simulink model "ES239A_HwAgCorrln"  (R2013b)
settings: Solver=FixedStepDiscrete  SolverMode=SingleTasking  StartTime=0.0  StopTime=1  FixedStep=0.002  RelTol=1e-3
values from neighbouring files (symbols this model uses):
  FLTINJ_HWAGCORRLN_HWAGIDPTSIG = DataDict.Constant    [ES239A_HwAgCorrln_DataDict.m]
  HwAgCorrlnHwAgAbsltDif = DataDict.Calibration    [ES239A_HwAgCorrln_DataDict.m]
  HwAgCorrlnHwAgMaxStall = DataDict.Calibration    [ES239A_HwAgCorrln_DataDict.m]
  HwAgCorrlnNtc0x092FailStep = DataDict.Calibration    [ES239A_HwAgCorrln_DataDict.m]
  HwAgCorrlnNtc0x092PassStep = DataDict.Calibration    [ES239A_HwAgCorrln_DataDict.m]
undefined symbols (not defined in the file or in its folder): NtcNr1, NtcSts1, sigbuilder_block
libraries: simulink x2, NxtrLim x2
(part 1 of 2)
settings Model: Creator=rzqy0r  LastModifiedBy=FZG88Y
settings SolverCC: AutoInsertRateTranBlk=on  InsertRTBMode=Always
settings DataIOCC: LimitDataPoints=off  SaveFormat=Structure  ReturnWorkspaceOutputs=on
settings OptimizationCC: BlockReduction=off  InlineParams=on  ZeroExternalMemoryAtStartup=off  ZeroInternalMemoryAtStartup=off  OptimizeModelRefInitCode=on  LifeSpan=1
settings DebuggingCC: SignalInfNanChecking=error  SignalRangeChecking=warning  UnderspecifiedInitializationDetection=Simplified  SolverPrmCheckMsg=error  InheritedTsInSrcMsg=error  DiscreteInheritContinuousMsg=error  SingleTaskRateTransMsg=error  TasksWithSamePriorityMsg=error  SigSpecEnsureSampleTimeMsg=error  CheckMatrixSingularityMsg=error  ParameterUnderflowMsg=error  ParameterPrecisionLossMsg=error  ParameterTunabilityLossMsg=error  FixptConstUnderflowMsg=warning  FixptConstOverflowMsg=warning  VectorMatrixConversionMsg=error  SignalLabelMismatchMsg=error  UnconnectedInputMsg=error  UnconnectedOutputMsg=error  UnconnectedLineMsg=error  SFcnCompatibilityMsg=error  UniqueDataStoreMsg=warning  BusObjectLabelMismatch=error  RootOutportRequireBusObject=error  AssertControl=DisableAll  ModelReferenceIOMsg=error  ModelReferenceVersionMismatchMessage=warning  ModelReferenceIOMismatchMessage=error  ModelReferenceCSMismatchMessage=warning  ModelReferenceDataLoggingMessage=error  StateNameClashWarn=warning  StrictBusMsg=ErrorOnBusTreatedAsVector  NonBusSignalsTreatedAsBus=error  SFUnexpectedBacktrackingDiag=error  SFInvalidInputDataAccessInChartInitDiag=error  SFNoUnconditionalDefaultTransitionDiag=error  SFTransitionOutsideNaturalParentDiag=error  SFUnconditionalTransitionShadowingDiag=error  SFUndirectedBroadcastEventsDiag=error
settings ModelReferenceCC: ModelReferenceNumInstancesAllowed=Single
settings RTWCC: SystemTargetFile=autosar.tlc  GenCodeOnly=on  TemplateMakefile=ert_default_tmf  Description=AUTOSAR  GenerateReport=on  ProcessScript=autosar_make_rtw_hook  LaunchReport=on
settings CodeAppCC: GenerateComments=off  IgnoreCustomStorageClasses=off  CustomSymbolStrType=$N$R$M  CustomSymbolStrBlkIO=$N$M  SimulinkBlockComments=off
settings STFCustomTargetCC: ParMdlRefBuildCompliant=on  CompOptLevelCompliant=on  IncludeMdlTerminateFcn=off  CombineOutputUpdateFcns=on  SuppressErrorStatus=on  ERTFirstTimeCompliant=on  ERTCustomFileBanners=on  SupportNonFinite=off  SupportComplex=off  SupportContinuousTime=off  SupportNonInlinedSFcns=off  MATLABClassNameForMDSCustomization=Simulink.SoftwareTarget.ERTCustomization  AutosarCompliant=on  GRTInterface=off  SystemTargetFile=autosar.tlc
settings ERTTargetCC: CodeReplacementLibrary=ANSI_C  ConcurrentExecutionCompliant=off  IncludeMdlTerminateFcn=off  SuppressErrorStatus=on  SupportNonFinite=off  SupportComplex=off  ModelStepFunctionPrototypeControlCompliant=off  CPPClassGenCompliant=off  AutosarCompliant=on  InlinedParameterPlacement=NonHierarchical  ERTCustomFileTemplate=example_file_process.tlc  EnableUserReplacementTypes=on

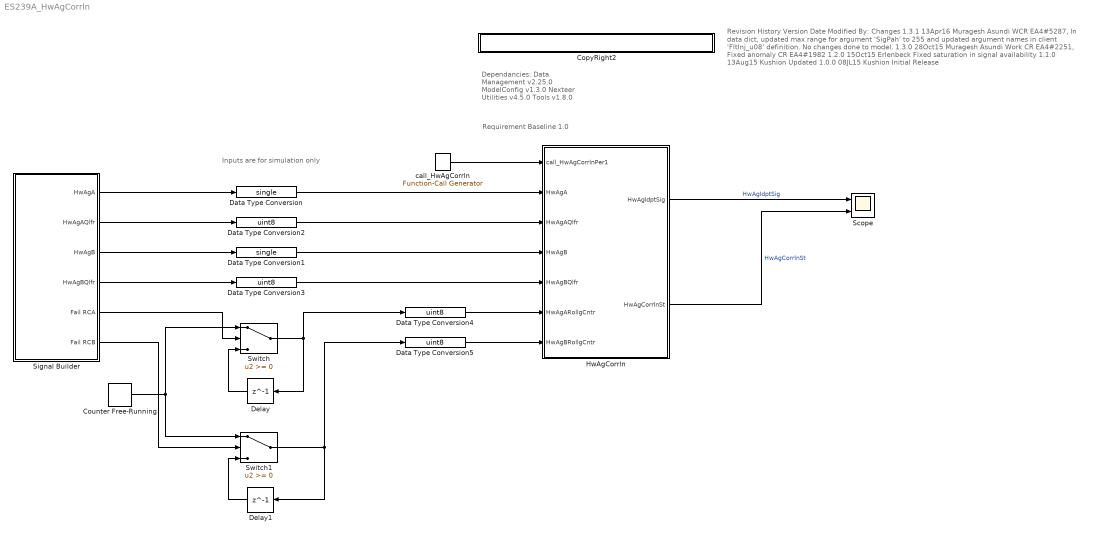
== system ES239A_HwAgCorrln ==
  note: Requirement Baseline 1.0
  note: Inputs are for simulation only
  note: Revision History
      |
      | Version		Date 		Modified By: 		Changes
      |
      | 1.3.1              13Apr16        Muragesh Asundi  WCR EA4#5287, In data dict, updated max range for argument 'SigPah' to 255 and updated argument names in client 'FltInj_u08' definition.
      |                                                                          No changes done to model.
      | 1.3.0              28Oct15        Muragesh Asundi  Work CR EA4#2251, Fixed anomaly CR EA4#1982
      | 1.2.0              15Oct15        Erlenbeck             Fixed saturation in signal availability
      | 1.1.0              13Aug15       Kushion                Updated
      | 1.0.0 		08JL15		Kushion			Initial Release
  note: Dependancies:
      |    Data Management v2.25.0
      |    ModelConfig v1.3.0
      |    Nexteer Utilities v4.5.0
      |    Tools v1.8.0
  CopyRight2 : Subsystem  Description=|  mask(Copyright Information){none=on}
      | Copyright info block.                                               
      |                                                                     
      | Place copyright information at the top of every subsystem in design.
      mask prompts: none "No parameters"
      mask help: Place copyright information at the top of every subsystem in design.
      mask Display:
      | NxtrConf = 'Nexteer Confidential';
      | 
      | sys = bdroot; %handle for the current model ("system")
      | first = get_param(sys,'Created');
      | first = first(end-3:end);  %year is last four digits
      | 
      | last = get_param(sys,'LastModifiedDate');
      | if isempty(last)
      |     last = datestr(now,'yyyy');
      | else
      |     last = last(end-3:end);
      | end
      | 
      | if strcmp(first,last)
      |     fprintf('%s -- Copyright %s Nexteer',NxtrConf,first)
      | else
      |     fprintf('%s -- %s%s- %s Nexteer',NxtrConf,char(169),first,last)
      | end
  Counter Free-Running : simulink/Sources/Counter Free-Running  NumBits=8  tsamp=0.004
  Data Type Conversion : DataTypeConversion  OutDataTypeStr=single
  Data Type Conversion1 : DataTypeConversion  OutDataTypeStr=single
  Data Type Conversion{2..5} (4 alike) : DataTypeConversion  OutDataTypeStr=uint8
  Delay : Delay  DelayLength=1  InitialCondition=0  SampleTime=0.004
  Delay1 : Delay  DelayLength=1  InitialCondition=0  SampleTime=0.004
  HwAgCorrln : Subsystem
      settings: AttributesFormatString=%<Tag>
  Scope : Scope  NumInputPorts=2
      settings: TimeRange=10  YMin=0~0  YMax=5~5  MaxDataPoints=10000
  Signal Builder : Subsystem  Tag=STV Subsys  LoadFcn=sigbuilder_block('load');  StartFcn=sigbuilder_block('start');  StopFcn=sigbuilder_block('stop');  ClipboardFcn=sigbuilder_block('clipboard');  mask(Sigbuilder block){}
      mask help: Simulink:masks:SigbuilderBlock_MD
      mask init:
      | if ~strcmp(get_param(bdroot(gcbh),'SimulationStatus'),'stopped') tuvar = sigbuilder_block('maskInit'); end
      settings: CopyFcn=sigbuilder_block('copy');  DeleteFcn=sigbuilder_block('delete');  ModelCloseFcn=sigbuilder_block('modelClose');  PreSaveFcn=sigbuilder_block('preSave');  PauseFcn=sigbuilder_block('pause');  ContinueFcn=sigbuilder_block('continue');  NameChangeFcn=sigbuilder_block('namechange');  OpenFcn=sigbuilder_block('open',[21.75 99 490.5 414 ]);  CloseFcn=sigbuilder_block('close');
      mask Display: plot(0, 0, 100, 100,[2, 2, 32, 32, 2], [68, 8, 8, 68, 68],[32, 2], [38, 38], [32, 19, 2],[53, 60, 44], [32, 17, 17, 2],[16, 16, 31, 31]);txt = getActiveGroup(gcbh);text(2, 100, txt,'verticalAlignment', 'top');
  Switch : Switch
  Switch1 : Switch
  call_HwAgCorrln : simulink/Ports & Subsystems/Function-Call Generator  sample_time=.004  numberOfIterations=1
  wires:
  call_HwAgCorrln/1 -> HwAgCorrln/1(call_HwAgCorrlnPer1)
  HwAgCorrln/1(HwAgIdptSig) -> Scope/1  "HwAgIdptSig"
  HwAgCorrln/2(HwAgCorrlnSt) -> Scope/2  "HwAgCorrlnSt"
  Signal Builder/5(Fail RCA) -> Switch/2
  Delay/1 -> Switch/3
  Switch/1 -> Delay/1, Data Type Conversion4/1
  Counter Free-Running/1 -> Switch1/1, Switch/1
  Signal Builder/6(Fail RCB) -> Switch1/2
  Delay1/1 -> Switch1/3
  Switch1/1 -> Data Type Conversion5/1, Delay1/1
  Signal Builder/1(HwAgA) -> Data Type Conversion/1
  Signal Builder/2(HwAgAQlfr) -> Data Type Conversion2/1
  Signal Builder/3(HwAgB) -> Data Type Conversion1/1
  Signal Builder/4(HwAgBQlfr) -> Data Type Conversion3/1
  Data Type Conversion1/1 -> HwAgCorrln/4(HwAgB)
  Data Type Conversion2/1 -> HwAgCorrln/3(HwAgAQlfr)
  Data Type Conversion3/1 -> HwAgCorrln/5(HwAgBQlfr)
  Data Type Conversion4/1 -> HwAgCorrln/6(HwAgARollgCntr)
  Data Type Conversion5/1 -> HwAgCorrln/7(HwAgBRollgCntr)
  Data Type Conversion/1 -> HwAgCorrln/2(HwAgA)

== system ES239A_HwAgCorrln/CopyRight2 ==

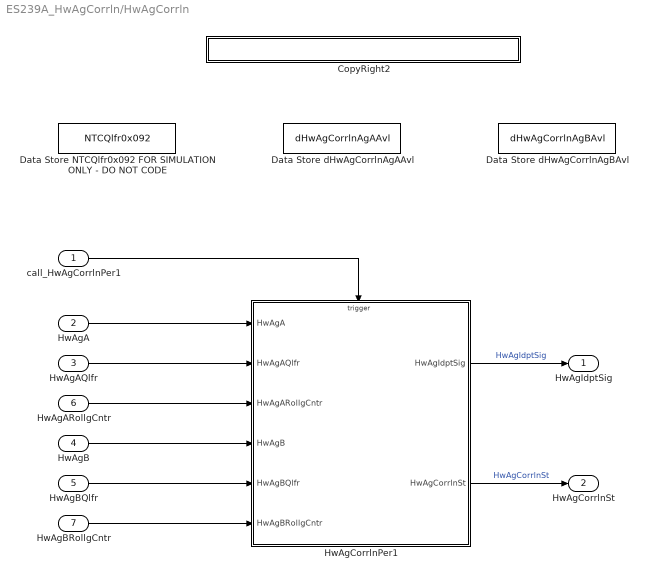
== system ES239A_HwAgCorrln/HwAgCorrln ==
  call_HwAgCorrlnPer1 : Inport
  HwAgA : Inport  Port=2
  HwAgAQlfr : Inport  Port=3
  HwAgB : Inport  Port=4
  HwAgBQlfr : Inport  Port=5
  HwAgARollgCntr : Inport  Port=6
  HwAgBRollgCntr : Inport  Port=7
  CopyRight2 : Subsystem  Description=|  mask(Copyright Information){none=on}
      | Copyright info block.                                               
      |                                                                     
      | Place copyright information at the top of every subsystem in design.
      mask prompts: none "No parameters"
      mask help: Place copyright information at the top of every subsystem in design.
      mask Display:
      | NxtrConf = 'Nexteer Confidential';
      | 
      | sys = bdroot; %handle for the current model ("system")
      | first = get_param(sys,'Created');
      | first = first(end-3:end);  %year is last four digits
      | 
      | last = get_param(sys,'LastModifiedDate');
      | if isempty(last)
      |     last = datestr(now,'yyyy');
      | else
      |     last = last(end-3:end);
      | end
      | 
      | if strcmp(first,last)
      |     fprintf('%s -- Copyright %s Nexteer',NxtrConf,first)
      | else
      |     fprintf('%s -- %s%s- %s Nexteer',NxtrConf,char(169),first,last)
      | end
  Data Store NTCQlfr0x092 FOR SIMULATION ONLY - DO NOT CODE : DataStoreMemory  DataStoreName=NTCQlfr0x092
  Data Store dHwAgCorrlnAgAAvl : DataStoreMemory  DataStoreName=dHwAgCorrlnAgAAvl
  Data Store dHwAgCorrlnAgBAvl : DataStoreMemory  DataStoreName=dHwAgCorrlnAgBAvl
  HwAgCorrlnPer1 : Subsystem  Tag=0.002  TreatAsAtomicUnit=on
  HwAgIdptSig : Outport
  HwAgCorrlnSt : Outport  Port=2
  wires:
  HwAgCorrlnPer1/1(HwAgIdptSig) -> HwAgIdptSig/1  "HwAgIdptSig"
  call_HwAgCorrlnPer1/1 -> HwAgCorrlnPer1/Trigger
  HwAgA/1 -> HwAgCorrlnPer1/1(HwAgA)
  HwAgAQlfr/1 -> HwAgCorrlnPer1/2(HwAgAQlfr)
  HwAgARollgCntr/1 -> HwAgCorrlnPer1/3(HwAgARollgCntr)
  HwAgB/1 -> HwAgCorrlnPer1/4(HwAgB)
  HwAgBQlfr/1 -> HwAgCorrlnPer1/5(HwAgBQlfr)
  HwAgBRollgCntr/1 -> HwAgCorrlnPer1/6(HwAgBRollgCntr)
  HwAgCorrlnPer1/2(HwAgCorrlnSt) -> HwAgCorrlnSt/1  "HwAgCorrlnSt"

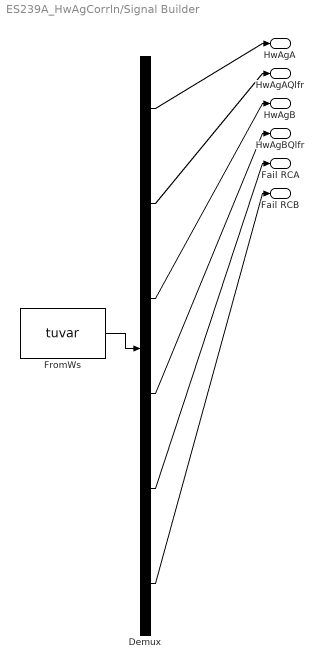
== system ES239A_HwAgCorrln/Signal Builder ==
  Demux : Demux  Tag=STV Demux  Outputs=6
  FromWs : FromWorkspace  Tag=STV FromWs  VariableName=tuvar  SampleTime=0
      SigBuilderData=|
      | common.afterFinalStr = 'Extrapolate'
      | common.sampleTime = 0
      | dataSet(1).timeRange = [0 10]
      | dataSet(1).name = 'Normal Op'
      | dataSet(2).timeRange = [0 10]
      | dataSet(2).name = 'Correlation Failure'
      | dataSet(3).timeRange = [0 10]
      | dataSet(3).name = 'Qualifier A Failure Hold Last Value with Recovery'
      | dataSet(4).timeRange = [0 10]
      | dataSet(4).name = 'Short Qualifier A Failure - Confirm immediate Status but no indpt reduction'
      | dataSet(5).timeRange = [0 10]
      | dataSet(5).name = 'Qualifier A and B Failure with recovery'
      | sbobj.Groups(1).Name = 'Normal Op'
      | sbobj.Groups(1).Signals(1).Name = 'HwAgA'
      | sbobj.Groups(1).Signals(1).XData = [0 1 2 3 4 5 6 7 8 9 10]
      | sbobj.Groups(1).Signals(1).YData = [0 900 -900 900 -900 900 -222 180 0 0 0]
      | sbobj.Groups(1).Signals(2).Name = 'HwAgAQlfr'
      | sbobj.Groups(1).Signals(2).XData = [0 0.8 0.8 6 10]
      | sbobj.Groups(1).Signals(2).YData = [0 0 1 1 1]
      | sbobj.Groups(1).Signals(3).Name = 'HwAgB'
      | sbobj.Groups(1).Signals(3).XData = [0 1 2 3 4 5 6 7 8 9 10]
      | sbobj.Groups(1).Signals(3).YData = [0 900 -900 900 -900 900 -222 180 0 0 0]
      | sbobj.Groups(1).Signals(4).Name = 'HwAgBQlfr'
      | sbobj.Groups(1).Signals(4).XData = [0 1 1 2 10]
      | sbobj.Groups(1).Signals(4).YData = [0 0 1 1 1]
      | sbobj.Groups(1).Signals(5).Name = 'Fail RCA'
      | sbobj.Groups(1).Signals(5).XData = [0 4 6 10]
      | sbobj.Groups(1).Signals(5).YData = [1 1 1 1]
      | sbobj.Groups(1).Signals(6).Name = 'Fail RCB'
      | sbobj.Groups(1).Signals(6).XData = [0 4 6 10]
      | sbobj.Groups(1).Signals(6).YData = [1 1 1 1]
      | sbobj.Groups(2).Name = 'Correlation Failure'
      | sbobj.Groups(2).Signals(1).Name = 'HwAgA'
      | sbobj.Groups(2).Signals(1).XData = [0 1 2 3 4 5 6 7 8 9 10]
      | sbobj.Groups(2).Signals(1).YData = [0 900 -900 900 -900 900 -222 180 0 0 0]
      | sbobj.Groups(2).Signals(2).Name = 'HwAgAQlfr'
      | sbobj.Groups(2).Signals(2).XData = [0 0.8 0.8 6 10]
      | sbobj.Groups(2).Signals(2).YData = [0 0 1 1 1]
      | sbobj.Groups(2).Signals(3).Name = 'HwAgB'
      | sbobj.Groups(2).Signals(3).XData = [0 1 2 3 4 5 6 7 8 9 10]
      | sbobj.Groups(2).Signals(3).YData = [0 900 -900 900 -900 900 -222 -264.9 0 0 0]
      | sbobj.Groups(2).Signals(4).Name = 'HwAgBQlfr'
      | sbobj.Groups(2).Signals(4).XData = [0 1 1 2 10]
      | sbobj.Groups(2).Signals(4).YData = [0 0 1 1 1]
      | sbobj.Groups(2).Signals(5).Name = 'Fail RCA'
      | sbobj.Groups(2).Signals(5).XData = [0 4 6 10]
      | sbobj.Groups(2).Signals(5).YData = [1 1 1 1]
      | sbobj.Groups(2).Signals(6).Name = 'Fail RCB'
      | sbobj.Groups(2).Signals(6).XData = [0 4 6 10]
      | sbobj.Groups(2).Signals(6).YData = [1 1 1 1]
      | sbobj.Groups(3).Name = 'Qualifier A Failure Hold Last Value with Recovery'
      | sbobj.Groups(3).Signals(1).Name = 'HwAgA'
      | sbobj.Groups(3).Signals(1).XData = [0 1 2 3 4 5 6 7 8 9 10]
      | sbobj.Groups(3).Signals(1).YData = [0 900 -900 900 -900 900 -222 180 0 0 0]
      | sbobj.Groups(3).Signals(2).Name = 'HwAgAQlfr'
      | sbobj.Groups(3).Signals(2).XData = [0 0.8 0.8 6 10]
      | sbobj.Groups(3).Signals(2).YData = [0 0 1 1 1]
      | sbobj.Groups(3).Signals(3).Name = 'HwAgB'
      | sbobj.Groups(3).Signals(3).XData = [0 1 2 3 4 5 5 6 7 8 9 10]
      | sbobj.Groups(3).Signals(3).YData = [0 900 -900 -900 -900 -900 900 -222 180 0 0 0]
      | sbobj.Groups(3).Signals(4).Name = 'HwAgBQlfr'
      | sbobj.Groups(3).Signals(4).XData = [0 1 1 2 2 3 4 5 5 10]
      | sbobj.Groups(3).Signals(4).YData = [0 0 1 1 2 2 2 2 1 1]
      | sbobj.Groups(3).Signals(5).Name = 'Fail RCA'
      | sbobj.Groups(3).Signals(5).XData = [0 4 6 10]
      | sbobj.Groups(3).Signals(5).YData = [1 1 1 1]
      | sbobj.Groups(3).Signals(6).Name = 'Fail RCB'
      | sbobj.Groups(3).Signals(6).XData = [0 4 6 10]
      | sbobj.Groups(3).Signals(6).YData = [1 1 1 1]
      | sbobj.Groups(4).Name = 'Short Qualifier A Failure - Confirm immediate Status but no indpt reduction'
      | sbobj.Groups(4).Signals(1).Name = 'HwAgA'
      | sbobj.Groups(4).Signals(1).XData = [0 1 2 3 4 5 6 7 8 9 10]
      | sbobj.Groups(4).Signals(1).YData = [0 900 -900 900 -900 900 -222 180 0 0 0]
      | sbobj.Groups(4).Signals(2).Name = 'HwAgAQlfr'
      | sbobj.Groups(4).Signals(2).XData = [0 0.8 0.8 6 10]
      | sbobj.Groups(4).Signals(2).YData = [0 0 1 1 1]
      | sbobj.Groups(4).Signals(3).Name = 'HwAgB'
      | sbobj.Groups(4).Signals(3).XData = [0 1 2 3 4 5 6 7 8 9 10]
      | sbobj.Groups(4).Signals(3).YData = [0 900 -900 900 -900 900 -222 180 0 0 0]
      | sbobj.Groups(4).Signals(4).Name = 'HwAgBQlfr'
      | sbobj.Groups(4).Signals(4).XData = [0 1 1 2 2 2.05 2.05 4 5 10]
      | sbobj.Groups(4).Signals(4).YData = [0 0 1 1 2 2 1 1 1 1]
      | sbobj.Groups(4).Signals(5).Name = 'Fail RCA'
      | sbobj.Groups(4).Signals(5).XData = [0 4 6 10]
      | sbobj.Groups(4).Signals(5).YData = [1 1 1 1]
      | sbobj.Groups(4).Signals(6).Name = 'Fail RCB'
      | sbobj.Groups(4).Signals(6).XData = [0 4 6 10]
      | sbobj.Groups(4).Signals(6).YData = [1 1 1 1]
      | sbobj.Groups(5).Name = 'Qualifier A and B Failure with recovery'
      | sbobj.Groups(5).Signals(1).Name = 'HwAgA'
      | sbobj.Groups(5).Signals(1).XData = [0 1 2 3 4 5 6 6 7 8 9 10]
      | sbobj.Groups(5).Signals(1).YData = [0 900 -900 900 -900 -900 -900 -222 180 0 0 0]
      | sbobj.Groups(5).Signals(2).Name = 'HwAgAQlfr'
      | sbobj.Groups(5).Signals(2).XData = [0 0.8 0.8 4 4 6 6 10]
      | sbobj.Groups(5).Signals(2).YData = [0 0 1 1 2 2 1 1]
      | sbobj.Groups(5).Signals(3).Name = 'HwAgB'
      | sbobj.Groups(5).Signals(3).XData = [0 1 2 3 4 5 5 6 7 8 9 10]
      | sbobj.Groups(5).Signals(3).YData = [0 900 -900 -900 -900 -900 900 -222 180 0 0 0]
      | sbobj.Groups(5).Signals(4).Name = 'HwAgBQlfr'
      | sbobj.Groups(5).Signals(4).XData = [0 1 1 2 2 3 4 5 5 10]
      | sbobj.Groups(5).Signals(4).YData = [0 0 1 1 2 2 2 2 1 1]
      | sbobj.Groups(5).Signals(5).Name = 'Fail RCA'
      | sbobj.Groups(5).Signals(5).XData = [0 4 6 10]
      | sbobj.Groups(5).Signals(5).YData = [1 1 1 1]
      | sbobj.Groups(5).Signals(6).Name = 'Fail RCB'
      | sbobj.Groups(5).Signals(6).XData = [0 4 6 10]
      | sbobj.Groups(5).Signals(6).YData = [1 1 1 1]
  HwAgA : Outport  Tag=STV Outport
  HwAgAQlfr : Outport  Tag=STV Outport  Port=2
  HwAgB : Outport  Tag=STV Outport  Port=3
  HwAgBQlfr : Outport  Tag=STV Outport  Port=4
  Fail RCA : Outport  Tag=STV Outport  Port=5
  Fail RCB : Outport  Tag=STV Outport  Port=6
  wires:
  FromWs/1 -> Demux/1
  Demux/1 -> HwAgA/1
  Demux/2 -> HwAgAQlfr/1
  Demux/3 -> HwAgB/1
  Demux/4 -> HwAgBQlfr/1
  Demux/5 -> Fail RCA/1
  Demux/6 -> Fail RCB/1

== system ES239A_HwAgCorrln/HwAgCorrln/CopyRight2 ==

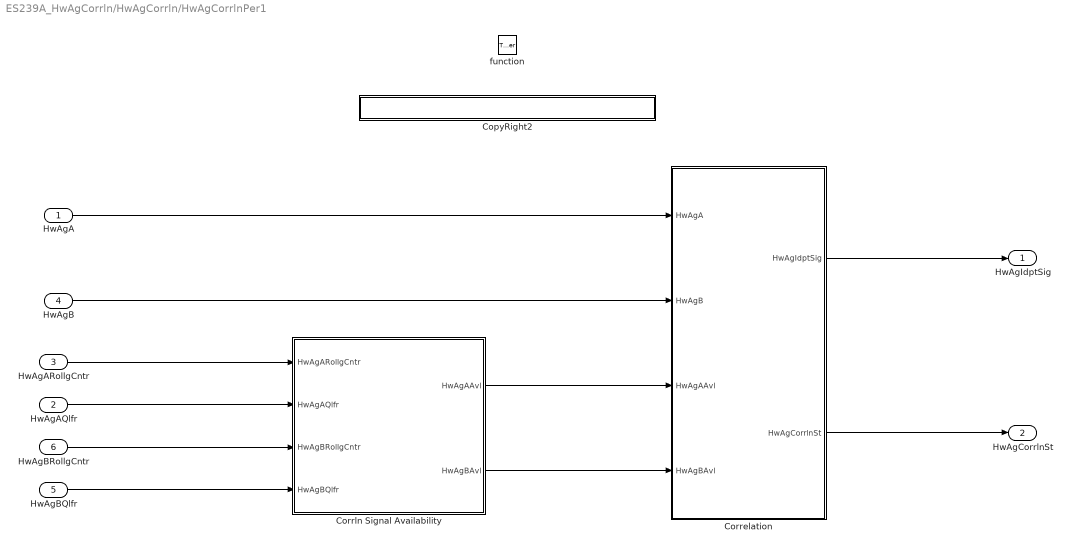
== system ES239A_HwAgCorrln/HwAgCorrln/HwAgCorrlnPer1 ==
  HwAgA : Inport
  HwAgAQlfr : Inport  Port=2
  HwAgARollgCntr : Inport  Port=3
  HwAgB : Inport  Port=4
  HwAgBQlfr : Inport  Port=5
  HwAgBRollgCntr : Inport  Port=6
  function : TriggerPort  TriggerType=function-call
  CopyRight2 : Subsystem  Description=|  mask(Copyright Information){none=on}
      | Copyright info block.                                               
      |                                                                     
      | Place copyright information at the top of every subsystem in design.
      mask prompts: none "No parameters"
      mask help: Place copyright information at the top of every subsystem in design.
      mask Display:
      | NxtrConf = 'Nexteer Confidential';
      | 
      | sys = bdroot; %handle for the current model ("system")
      | first = get_param(sys,'Created');
      | first = first(end-3:end);  %year is last four digits
      | 
      | last = get_param(sys,'LastModifiedDate');
      | if isempty(last)
      |     last = datestr(now,'yyyy');
      | else
      |     last = last(end-3:end);
      | end
      | 
      | if strcmp(first,last)
      |     fprintf('%s -- Copyright %s Nexteer',NxtrConf,first)
      | else
      |     fprintf('%s -- %s%s- %s Nexteer',NxtrConf,char(169),first,last)
      | end
  "Correlation " : Subsystem
  Corrln Signal Availability : Subsystem
  HwAgIdptSig : Outport
  HwAgCorrlnSt : Outport  Port=2
  wires:
  HwAgAQlfr/1 -> Corrln Signal Availability/2(HwAgAQlfr)
  HwAgARollgCntr/1 -> Corrln Signal Availability/1(HwAgARollgCntr)
  HwAgBQlfr/1 -> Corrln Signal Availability/4(HwAgBQlfr)
  HwAgBRollgCntr/1 -> Corrln Signal Availability/3(HwAgBRollgCntr)
  HwAgA/1 -> "Correlation "/1(HwAgA)
  HwAgB/1 -> "Correlation "/2(HwAgB)
  "Correlation "/1(HwAgIdptSig) -> HwAgIdptSig/1
  "Correlation "/2(HwAgCorrlnSt) -> HwAgCorrlnSt/1
  Corrln Signal Availability/1(HwAgAAvl) -> "Correlation "/3(HwAgAAvl)
  Corrln Signal Availability/2(HwAgBAvl) -> "Correlation "/4(HwAgBAvl)

== system ES239A_HwAgCorrln/HwAgCorrln/HwAgCorrlnPer1/CopyRight2 ==

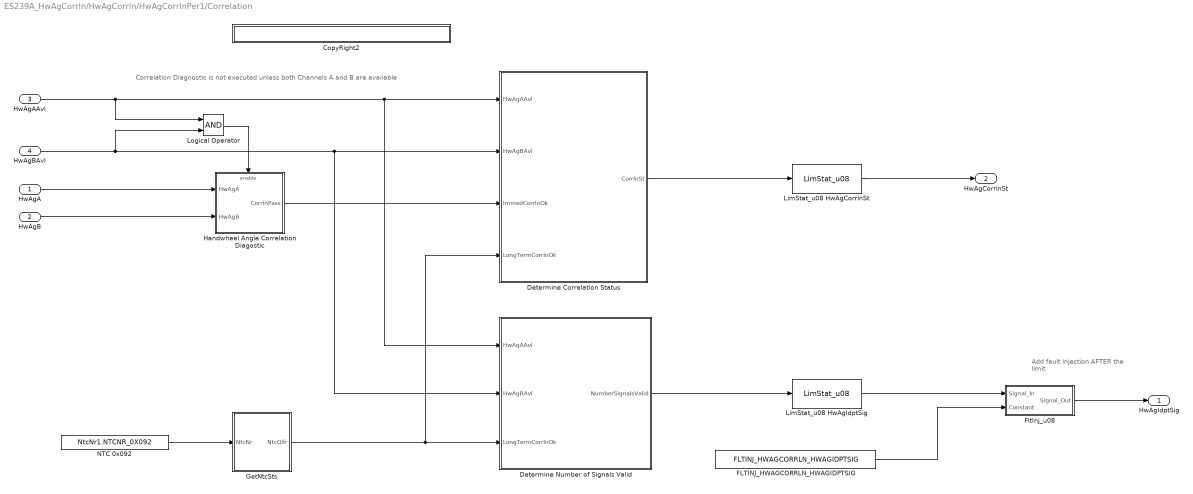
== system ES239A_HwAgCorrln/HwAgCorrln/HwAgCorrlnPer1/Correlation  ==
  note: Add fault injection
      | AFTER the limit
  note: Correlation Diagnostic is not executed unless both Channels A and B are available
  HwAgA : Inport
  HwAgB : Inport  Port=2
  HwAgAAvl : Inport  Port=3
  HwAgBAvl : Inport  Port=4
  CopyRight2 : Subsystem  Description=|  mask(Copyright Information){none=on}
      | Copyright info block.                                               
      |                                                                     
      | Place copyright information at the top of every subsystem in design.
      mask prompts: none "No parameters"
      mask help: Place copyright information at the top of every subsystem in design.
      mask Display:
      | NxtrConf = 'Nexteer Confidential';
      | 
      | sys = bdroot; %handle for the current model ("system")
      | first = get_param(sys,'Created');
      | first = first(end-3:end);  %year is last four digits
      | 
      | last = get_param(sys,'LastModifiedDate');
      | if isempty(last)
      |     last = datestr(now,'yyyy');
      | else
      |     last = last(end-3:end);
      | end
      | 
      | if strcmp(first,last)
      |     fprintf('%s -- Copyright %s Nexteer',NxtrConf,first)
      | else
      |     fprintf('%s -- %s%s- %s Nexteer',NxtrConf,char(169),first,last)
      | end
  Determine Correlation Status : Truth Table  RequirementInfo={'linktype_rmi_doors' '0000cf63 (/E-STEER Core/SubSystem Specifications/Electrical Actuator/Control Module/FDD Module Requirements/EA4/ES239A_HwAgCorrl_Draft)' '#ES239A_100' 'true' 'REQ: ES239A_100' '' ; 'linktype_rmi_doors' '0000cf63 (/E-STEER Core/SubSystem Specifications/Electrical Actuator/Control Module/FDD Module Requirements/EA4/ES239A_HwAgCorrl_Draft)' '#ES239A_109' 'true' 'REQ: ES239A_109' '' ; 'linktype_rmi_doors' '0000cf63 (/E-STEER Core/SubSystem Specifications/Electrical Actuator/Control Module/FDD Module Requirements/EA4/ES239A_HwAgCorrl_Draft)' '#ES239A_110' 'true' 'REQ: ES239A_110' '' ; 'linktype_rmi_doors' '0000cf63 (/E-STEER Core/SubSystem Specifications/Electrical Actuator/Control Module/FDD Module Requirements/EA4/ES239A_HwAgCorrl_Draft)' '#ES239A_112' 'true' 'REQ: ES239A_112' '' ; 'linktype_rmi_doors' '0000cf63 (/E-STEER Core/SubSystem Specifications/Electrical Actuator/Control Module/FDD Module Requirements/EA4/ES239A_HwAgCorrl_Draft)' '#ES239A_113' 'true' 'REQ: ES239A_113' '' } %GIDa_67b947a1_7168_4e60_a621_20ab2a82f9e4  TreatAsAtomicUnit=on
  Determine Number of Signals Valid : Truth Table  RequirementInfo={'linktype_rmi_doors' '0000cf63 (/E-STEER Core/SubSystem Specifications/Electrical Actuator/Control Module/FDD Module Requirements/EA4/ES239A_HwAgCorrl_Draft)' '#ES239A_119' 'true' 'REQ: ES239A_119' '' ; 'linktype_rmi_doors' '0000cf63 (/E-STEER Core/SubSystem Specifications/Electrical Actuator/Control Module/FDD Module Requirements/EA4/ES239A_HwAgCorrl_Draft)' '#ES239A_129' 'true' 'REQ: ES239A_129' '' ; 'linktype_rmi_doors' '0000cf63 (/E-STEER Core/SubSystem Specifications/Electrical Actuator/Control Module/FDD Module Requirements/EA4/ES239A_HwAgCorrl_Draft)' '#ES239A_124' 'true' 'REQ: ES239A_124' '' ; 'linktype_rmi_doors' '0000cf63 (/E-STEER Core/SubSystem Specifications/Electrical Actuator/Control Module/FDD Module Requirements/EA4/ES239A_HwAgCorrl_Draft)' '#ES239A_120' 'true' 'REQ: ES239A_120' '' ; 'linktype_rmi_doors' '0000cf63 (/E-STEER Core/SubSystem Specifications/Electrical Actuator/Control Module/FDD Module Requirements/EA4/ES239A_HwAgCorrl_Draft)' '#ES239A_122' 'true' 'REQ: ES239A_122' '' } %GIDa_35106513_c3c0_4da1_834f_7379f79731d2  TreatAsAtomicUnit=on
  FLTINJ_HWAGCORRLN_HWAGIDPTSIG : Constant  RequirementInfo={'linktype_rmi_doors' '0000cf63 (/E-STEER Core/SubSystem Specifications/Electrical Actuator/Control Module/FDD Module Requirements/EA4/ES239A_HwAgCorrl_Draft)' '#ES239A_139' 'true' 'REQ: ES239A_139' '' } %GIDa_dcd4ef43_6b76_41ba_bfae_1fba77b8b422  Value=FLTINJ_HWAGCORRLN_HWAGIDPTSIG
  FltInj_u08 : Subsystem  RequirementInfo={'linktype_rmi_doors' '0000cf63 (/E-STEER Core/SubSystem Specifications/Electrical Actuator/Control Module/FDD Module Requirements/EA4/ES239A_HwAgCorrl)' '#ES239A_139' 'true' 'REQ: ES239A_139' '' } %GIDa_81dbf112_3f37_469e_8630_4577ca85f452  TreatAsAtomicUnit=on  VariantControl=FltInj_sim  mask(Fault_Injection){}
      mask help: Fault Injection is a simulation only block for EA3 programs.
  GetNtcSts : Subsystem  RequirementInfo="{'linktype_rmi_doors' '000089e3 (/E-STEER_New/System Specification Documents/Core Specs/Subsystem Specs/System Functions FDD/SF-46  Gross Cross Check)' '#216' 'true' 'REQ: SF046A_216' '' ; 'linktype_rmi_doors' '000089e3 (/E-STEER_New/System Specification Documents/Core Specs/Subsystem Specs/System Functions FDD/SF-46  Gross Cross Check)' '#194' 'true' 'REQ: SF046A_194' '' } %GIDa_ef1d6f8b_71e6_4818_8330_18930fdabeca"  TreatAsAtomicUnit=on  mask(GetNTC){}
      mask help: GetNTC library block
      settings: RTWSystemCode=Inline
  "Handwheel Angle Correlation Diagostic " : Subsystem
  LimStat_u08 HwAgCorrlnSt : NxtrLim/LimStat_u08  LoLim=CORRLNSTSMINVAL_CNT_U08  HiLim=CORRLNSTSMAXVAL_CNT_U08
      settings: AttributesFormatString=|
      | Low Limit: %<LoLim>
      | High Limit:%<HiLim>
  LimStat_u08 HwAgIdptSig : NxtrLim/LimStat_u08  LoLim=NRVLDSIGMIN_CNT_U08  HiLim=NRVLDSIGMAX_CNT_U08
      settings: AttributesFormatString=|
      | Low Limit: %<LoLim>
      | High Limit:%<HiLim>
  Logical Operator : Logic  RequirementInfo={'linktype_rmi_doors' '0000cf63 (/E-STEER Core/SubSystem Specifications/Electrical Actuator/Control Module/FDD Module Requirements/EA4/ES239A_HwAgCorrl_Draft)' '#ES239A_89' 'true' 'REQ: ES239A_89' '' } %GIDa_51757cff_8670_44c7_a486_bbfc48183997  AllPortsSameDT=off  OutDataTypeStr=boolean
  NTC 0x092 : Constant  RequirementInfo={} %GIDa_c4c7739a_112c_43ae_a6d7_ac3eaefc7378  Value=NtcNr1.NTCNR_0X092
  HwAgIdptSig : Outport
  HwAgCorrlnSt : Outport  Port=2
  wires:
  HwAgB/1 -> "Handwheel Angle Correlation Diagostic "/2(HwAgB)
  HwAgA/1 -> "Handwheel Angle Correlation Diagostic "/1(HwAgA)
  LimStat_u08 HwAgIdptSig/1 -> FltInj_u08/1(Signal_In)
  HwAgBAvl/1 -> Determine Number of Signals Valid/2(HwAgBAvl), Determine Correlation Status/2(HwAgBAvl), Logical Operator/2
  LimStat_u08 HwAgCorrlnSt/1 -> HwAgCorrlnSt/1
  HwAgAAvl/1 -> Determine Number of Signals Valid/1(HwAgAAvl), Determine Correlation Status/1(HwAgAAvl), Logical Operator/1
  GetNtcSts/1(NtcQlfr) -> Determine Correlation Status/4(LongTermCorrlnOk), Determine Number of Signals Valid/3(LongTermCorrlnOk)
  "Handwheel Angle Correlation Diagostic "/1(CorrlnPass) -> Determine Correlation Status/3(ImmedCorrlnOk)
  Logical Operator/1 -> "Handwheel Angle Correlation Diagostic "/Enable
  NTC 0x092/1 -> GetNtcSts/1(NtcNr)
  FltInj_u08/1(Signal_Out) -> HwAgIdptSig/1
  Determine Number of Signals Valid/1(NumberSignalsValid) -> LimStat_u08 HwAgIdptSig/1
  Determine Correlation Status/1(CorrlnSt) -> LimStat_u08 HwAgCorrlnSt/1
  FLTINJ_HWAGCORRLN_HWAGIDPTSIG/1 -> FltInj_u08/2(Constant)

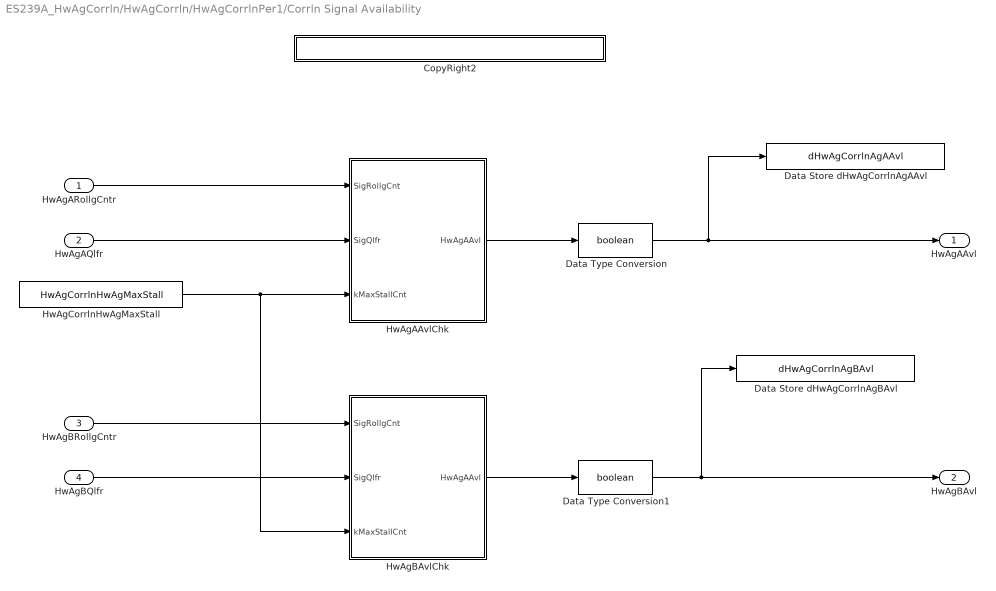
== system ES239A_HwAgCorrln/HwAgCorrln/HwAgCorrlnPer1/Corrln Signal Availability ==
  HwAgARollgCntr : Inport
  HwAgAQlfr : Inport  Port=2
  HwAgBRollgCntr : Inport  Port=3
  HwAgBQlfr : Inport  Port=4
  CopyRight2 : Subsystem  Description=|  mask(Copyright Information){none=on}
      | Copyright info block.                                               
      |                                                                     
      | Place copyright information at the top of every subsystem in design.
      mask prompts: none "No parameters"
      mask help: Place copyright information at the top of every subsystem in design.
      mask Display:
      | NxtrConf = 'Nexteer Confidential';
      | 
      | sys = bdroot; %handle for the current model ("system")
      | first = get_param(sys,'Created');
      | first = first(end-3:end);  %year is last four digits
      | 
      | last = get_param(sys,'LastModifiedDate');
      | if isempty(last)
      |     last = datestr(now,'yyyy');
      | else
      |     last = last(end-3:end);
      | end
      | 
      | if strcmp(first,last)
      |     fprintf('%s -- Copyright %s Nexteer',NxtrConf,first)
      | else
      |     fprintf('%s -- %s%s- %s Nexteer',NxtrConf,char(169),first,last)
      | end
  Data Store dHwAgCorrlnAgAAvl : DataStoreWrite  RequirementInfo={'linktype_rmi_doors' '0000cf63 (/E-STEER Core/SubSystem Specifications/Electrical Actuator/Control Module/FDD Module Requirements/EA4/ES239A_HwAgCorrl_Draft)' '#ES239A_140' 'true' 'REQ: ES239A_140' '' } %GIDa_69226d58_3222_4378_b58d_6edad87bfcb0  DataStoreName=dHwAgCorrlnAgAAvl
  Data Store dHwAgCorrlnAgBAvl : DataStoreWrite  RequirementInfo={'linktype_rmi_doors' '0000cf63 (/E-STEER Core/SubSystem Specifications/Electrical Actuator/Control Module/FDD Module Requirements/EA4/ES239A_HwAgCorrl_Draft)' '#ES239A_140' 'true' 'REQ: ES239A_140' '' } %GIDa_6b136ef5_51ed_463e_9439_42200f2ab483  DataStoreName=dHwAgCorrlnAgBAvl
  Data Type Conversion : DataTypeConversion  OutDataTypeStr=boolean
  Data Type Conversion1 : DataTypeConversion  OutDataTypeStr=boolean
  HwAgAAvlChk : Subsystem  RequirementInfo={'linktype_rmi_doors' '0000cf63 (/E-STEER Core/SubSystem Specifications/Electrical Actuator/Control Module/FDD Module Requirements/EA4/ES239A_HwAgCorrl_Draft)' '#ES239A_35' 'true' 'REQ: ES239A_35' '' } %GIDa_afd08659_04a6_48fb_a6d8_df09dfc0c7b5  TreatAsAtomicUnit=on
  HwAgBAvlChk : Subsystem  RequirementInfo={'linktype_rmi_doors' '0000cf63 (/E-STEER Core/SubSystem Specifications/Electrical Actuator/Control Module/FDD Module Requirements/EA4/ES239A_HwAgCorrl_Draft)' '#ES239A_69' 'true' 'REQ: ES239A_69' '' } %GIDa_d14d6223_2e9f_4d0d_b089_aec8048a6900  TreatAsAtomicUnit=on
  HwAgCorrlnHwAgMaxStall : Constant  Value=HwAgCorrlnHwAgMaxStall
  HwAgAAvl : Outport
  HwAgBAvl : Outport  Port=2
  wires:
  HwAgAQlfr/1 -> HwAgAAvlChk/2(SigQlfr)
  HwAgARollgCntr/1 -> HwAgAAvlChk/1(SigRollgCnt)
  HwAgBAvlChk/1(HwAgAAvl) -> Data Type Conversion1/1
  HwAgAAvlChk/1(HwAgAAvl) -> Data Type Conversion/1
  HwAgBRollgCntr/1 -> HwAgBAvlChk/1(SigRollgCnt)
  HwAgBQlfr/1 -> HwAgBAvlChk/2(SigQlfr)
  HwAgCorrlnHwAgMaxStall/1 -> HwAgBAvlChk/3(kMaxStallCnt), HwAgAAvlChk/3(kMaxStallCnt)
  Data Type Conversion/1 -> Data Store dHwAgCorrlnAgAAvl/1, HwAgAAvl/1
  Data Type Conversion1/1 -> Data Store dHwAgCorrlnAgBAvl/1, HwAgBAvl/1

== system ES239A_HwAgCorrln/HwAgCorrln/HwAgCorrlnPer1/Correlation /CopyRight2 ==

== system ES239A_HwAgCorrln/HwAgCorrln/HwAgCorrlnPer1/Correlation /FltInj_u08 ==
  note: This block requires no modification by FDD author.
      |
      | This block does not actually simulate any fault injection.  It is simply a pass-thru.
      |
      | The Constant port (#2) simply terminates its signal, but we are trying to force the FDD author
      | to properly use the FltInjectionLocType enumeration in FDD model.
  note: EA4.x Fault Injection
  Signal_In : Inport
  Constant : Inport  Port=2
  CopyRight2 : Subsystem  Description=|  mask(Copyright Information){none=on}
      | Copyright info block.                                               
      |                                                                     
      | Place copyright information at the top of every subsystem in design.
      mask prompts: none "No parameters"
      mask help: Place copyright information at the top of every subsystem in design.
      mask Display:
      | NxtrConf = 'Nexteer Confidential';
      | 
      | sys = bdroot; %handle for the current model ("system")
      | first = get_param(sys,'Created');
      | first = first(end-3:end);  %year is last four digits
      | 
      | last = get_param(sys,'LastModifiedDate');
      | if isempty(last)
      |     last = datestr(now,'yyyy');
      | else
      |     last = last(end-3:end);
      | end
      | 
      | if strcmp(first,last)
      |     fprintf('%s -- Copyright %s Nexteer',NxtrConf,first)
      | else
      |     fprintf('%s -- %s%s- %s Nexteer',NxtrConf,char(169),first,last)
      | end
  Terminator : Terminator
  Signal_Out : Outport
  wires:
  Signal_In/1 -> Signal_Out/1
  Constant/1 -> Terminator/1

== system ES239A_HwAgCorrln/HwAgCorrln/HwAgCorrlnPer1/Correlation /GetNtcSts ==
  NtcNr : Inport
  CopyRight2 : Subsystem  Description=|  mask(Copyright Information){none=on}
      | Copyright info block.                                               
      |                                                                     
      | Place copyright information at the top of every subsystem in design.
      mask prompts: none "No parameters"
      mask help: Place copyright information at the top of every subsystem in design.
      mask Display:
      | NxtrConf = 'Nexteer Confidential';
      | 
      | sys = bdroot; %handle for the current model ("system")
      | first = get_param(sys,'Created');
      | first = first(end-3:end);  %year is last four digits
      | 
      | last = get_param(sys,'LastModifiedDate');
      | if isempty(last)
      |     last = datestr(now,'yyyy');
      | else
      |     last = last(end-3:end);
      | end
      | 
      | if strcmp(first,last)
      |     fprintf('%s -- Copyright %s Nexteer',NxtrConf,first)
      | else
      |     fprintf('%s -- %s%s- %s Nexteer',NxtrConf,char(169),first,last)
      | end
  Data Store Read : DataStoreRead  DataStoreName=NTCQlfr0x092
  Terminator : Terminator
  NtcQlfr : Outport
  wires:
  NtcNr/1 -> Terminator/1
  Data Store Read/1 -> NtcQlfr/1

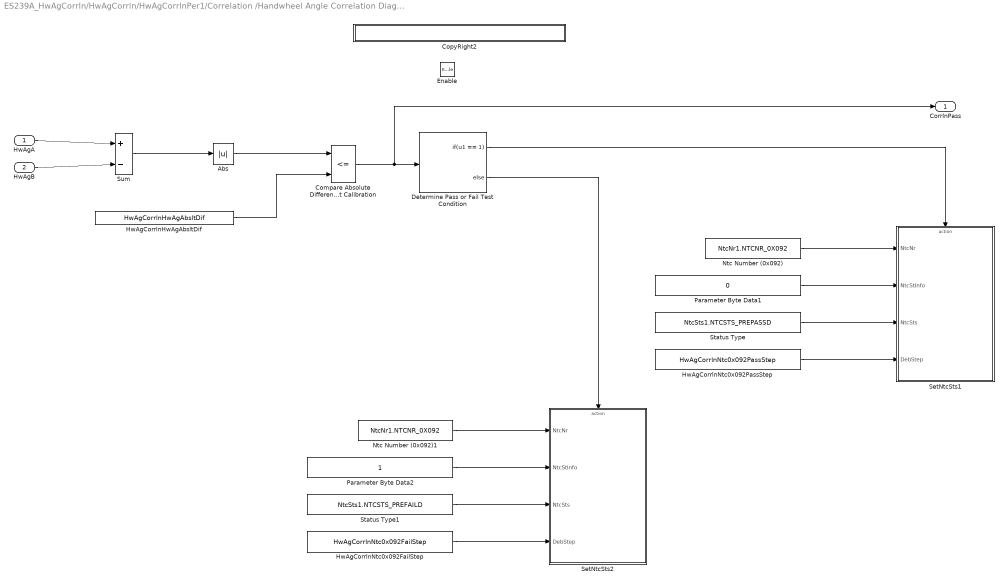
== system ES239A_HwAgCorrln/HwAgCorrln/HwAgCorrlnPer1/Correlation /Handwheel Angle Correlation Diagostic  ==
  HwAgA : Inport
  HwAgB : Inport  Port=2
  Enable : EnablePort
  Abs : Abs  RequirementInfo={'linktype_rmi_doors' '0000cf63 (/E-STEER Core/SubSystem Specifications/Electrical Actuator/Control Module/FDD Module Requirements/EA4/ES239A_HwAgCorrl_Draft)' '#ES239A_91' 'true' 'REQ: ES239A_91' '' } %GIDa_d3667a1c_f1b4_4f12_9455_ada967a0d26b
  Compare Absolute Difference Against Calibration : RelationalOperator  RequirementInfo={'linktype_rmi_doors' '0000cf63 (/E-STEER Core/SubSystem Specifications/Electrical Actuator/Control Module/FDD Module Requirements/EA4/ES239A_HwAgCorrl_Draft)' '#ES239A_91' 'true' 'REQ: ES239A_91' '' } %GIDa_0bf62408_cb2d_42db_92af_ff5b413c366f  Operator=<=  OutDataTypeStr=boolean
  CopyRight2 : Subsystem  Description=|  mask(Copyright Information){none=on}
      | Copyright info block.                                               
      |                                                                     
      | Place copyright information at the top of every subsystem in design.
      mask prompts: none "No parameters"
      mask help: Place copyright information at the top of every subsystem in design.
      mask Display:
      | NxtrConf = 'Nexteer Confidential';
      | 
      | sys = bdroot; %handle for the current model ("system")
      | first = get_param(sys,'Created');
      | first = first(end-3:end);  %year is last four digits
      | 
      | last = get_param(sys,'LastModifiedDate');
      | if isempty(last)
      |     last = datestr(now,'yyyy');
      | else
      |     last = last(end-3:end);
      | end
      | 
      | if strcmp(first,last)
      |     fprintf('%s -- Copyright %s Nexteer',NxtrConf,first)
      | else
      |     fprintf('%s -- %s%s- %s Nexteer',NxtrConf,char(169),first,last)
      | end
  Determine Pass or Fail Test Condition : If  RequirementInfo={'linktype_rmi_doors' '0000cf63 (/E-STEER Core/SubSystem Specifications/Electrical Actuator/Control Module/FDD Module Requirements/EA4/ES239A_HwAgCorrl_Draft)' '#ES239A_91' 'true' 'REQ: ES239A_91' '' } %GIDa_e9f56f03_4b0f_48e8_9036_e8c2bc5a328a  IfExpression=u1 == 1
  HwAgCorrlnHwAgAbsltDif : Constant  RequirementInfo={'linktype_rmi_doors' '0000cf63 (/E-STEER Core/SubSystem Specifications/Electrical Actuator/Control Module/FDD Module Requirements/EA4/ES239A_HwAgCorrl_Draft)' '#ES239A_91' 'true' 'REQ: ES239A_91' '' } %GIDa_2ab622e4_d24c_47f5_9327_6becf88fbd40  Value=HwAgCorrlnHwAgAbsltDif
  HwAgCorrlnNtc0x092FailStep : Constant  Value=HwAgCorrlnNtc0x092FailStep
  HwAgCorrlnNtc0x092PassStep : Constant  Value=HwAgCorrlnNtc0x092PassStep
  Ntc Number (0x092) : Constant  RequirementInfo={} %GIDa_7a38b9a3_2a93_479a_af17_083e50b2ad8e  Value=NtcNr1.NTCNR_0X092
  Ntc Number (0x092)1 : Constant  RequirementInfo={} %GIDa_d9866428_8d06_4f1e_bc40_884cb850d039  Value=NtcNr1.NTCNR_0X092
  Parameter Byte Data1 : Constant  Value=0  OutDataTypeStr=uint8
  Parameter Byte Data2 : Constant  OutDataTypeStr=uint8
  SetNtcSts1 : Subsystem  RequirementInfo={'linktype_rmi_doors' '0000cf63 (/E-STEER Core/SubSystem Specifications/Electrical Actuator/Control Module/FDD Module Requirements/EA4/ES239A_HwAgCorrl_Draft)' '#ES239A_94' 'true' 'REQ: ES239A_94' '' } %GIDa_817259c1_c1ab_4072_8765_1a611cdae0b3  mask(SetNTC){}
      mask help: SetNTC library block
  SetNtcSts2 : Subsystem  RequirementInfo={'linktype_rmi_doors' '0000cf63 (/E-STEER Core/SubSystem Specifications/Electrical Actuator/Control Module/FDD Module Requirements/EA4/ES239A_HwAgCorrl_Draft)' '#ES239A_91' 'true' 'REQ: ES239A_91' '' } %GIDa_65006a7c_ceba_4cc3_af6d_b38fbefcdc91  mask(SetNTC){}
      mask help: SetNTC library block
  Status Type : Constant  Value=NtcSts1.NTCSTS_PREPASSD
  Status Type1 : Constant  Value=NtcSts1.NTCSTS_PREFAILD
  Sum : Sum  RequirementInfo={'linktype_rmi_doors' '0000cf63 (/E-STEER Core/SubSystem Specifications/Electrical Actuator/Control Module/FDD Module Requirements/EA4/ES239A_HwAgCorrl_Draft)' '#ES239A_91' 'true' 'REQ: ES239A_91' '' } %GIDa_dcc5dc63_9e7f_483c_8b6e_6655a4583ac3  Inputs=+|-
  CorrlnPass : Outport
  wires:
  Sum/1 -> Abs/1
  HwAgB/1 -> Sum/2
  HwAgA/1 -> Sum/1
  Abs/1 -> Compare Absolute Difference Against Calibration/1
  HwAgCorrlnHwAgAbsltDif/1 -> Compare Absolute Difference Against Calibration/2
  Determine Pass or Fail Test Condition/1 -> SetNtcSts1/Action
  Determine Pass or Fail Test Condition/2 -> SetNtcSts2/Action
  Compare Absolute Difference Against Calibration/1 -> CorrlnPass/1, Determine Pass or Fail Test Condition/1
  Ntc Number (0x092)/1 -> SetNtcSts1/1(NtcNr)
  HwAgCorrlnNtc0x092PassStep/1 -> SetNtcSts1/4(DebStep)
  Status Type/1 -> SetNtcSts1/3(NtcSts)
  Parameter Byte Data1/1 -> SetNtcSts1/2(NtcStInfo)
  Ntc Number (0x092)1/1 -> SetNtcSts2/1(NtcNr)
  HwAgCorrlnNtc0x092FailStep/1 -> SetNtcSts2/4(DebStep)
  Status Type1/1 -> SetNtcSts2/3(NtcSts)
  Parameter Byte Data2/1 -> SetNtcSts2/2(NtcStInfo)

== system ES239A_HwAgCorrln/HwAgCorrln/HwAgCorrlnPer1/Corrln Signal Availability/CopyRight2 ==

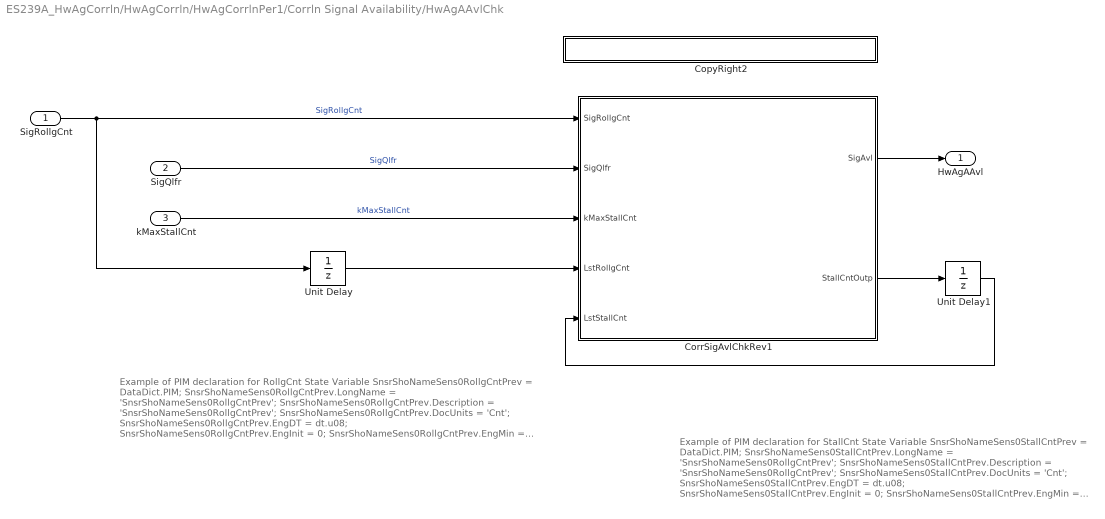
== system ES239A_HwAgCorrln/HwAgCorrln/HwAgCorrlnPer1/Corrln Signal Availability/HwAgAAvlChk ==
  note: Example of PIM declaration for StallCnt State Variable
      |
      | SnsrShoNameSens0StallCntPrev = DataDict.PIM;
      | SnsrShoNameSens0StallCntPrev.LongName = 'SnsrShoNameSens0RollgCntPrev';
      | SnsrShoNameSens0StallCntPrev.Description = 'SnsrShoNameSens0RollgCntPrev';
      | SnsrShoNameSens0StallCntPrev.DocUnits = 'Cnt';
      | SnsrShoNameSens0StallCntPrev.EngDT = dt.u08;
      | SnsrShoNameSens0StallCntPrev.EngInit = 0;
      | SnsrShoNameSens0StallCntPrev.EngMin = 0;
      | SnsrShoNameSens0StallCntPrev.EngMax = 255;
      |
      |
      | *********  Need different state variable for each instance of this  subsystem ********
  note: Example of PIM declaration for RollgCnt State Variable
      |
      | SnsrShoNameSens0RollgCntPrev = DataDict.PIM;
      | SnsrShoNameSens0RollgCntPrev.LongName = 'SnsrShoNameSens0RollgCntPrev';
      | SnsrShoNameSens0RollgCntPrev.Description = 'SnsrShoNameSens0RollgCntPrev';
      | SnsrShoNameSens0RollgCntPrev.DocUnits = 'Cnt';
      | SnsrShoNameSens0RollgCntPrev.EngDT = dt.u08;
      | SnsrShoNameSens0RollgCntPrev.EngInit = 0;
      | SnsrShoNameSens0RollgCntPrev.EngMin = 0;
      | SnsrShoNameSens0RollgCntPrev.EngMax = 255;
      |
      |
      | *********  Need different state variable for each instance of this  subsystem ********
  SigRollgCnt : Inport  OutDataTypeStr=uint8
  SigQlfr : Inport  Port=2  OutDataTypeStr=uint8
  kMaxStallCnt : Inport  Port=3  OutDataTypeStr=uint8
  CopyRight2 : Subsystem  Description=|  mask(Copyright Information){none=on}
      | Copyright info block.                                               
      |                                                                     
      | Place copyright information at the top of every subsystem in design.
      mask prompts: none "No parameters"
      mask help: Place copyright information at the top of every subsystem in design.
      mask Display:
      | NxtrConf = 'Nexteer Confidential';
      | 
      | sys = bdroot; %handle for the current model ("system")
      | first = get_param(sys,'Created');
      | first = first(end-3:end);  %year is last four digits
      | 
      | last = get_param(sys,'LastModifiedDate');
      | if isempty(last)
      |     last = datestr(now,'yyyy');
      | else
      |     last = last(end-3:end);
      | end
      | 
      | if strcmp(first,last)
      |     fprintf('%s -- Copyright %s Nexteer',NxtrConf,first)
      | else
      |     fprintf('%s -- %s%s- %s Nexteer',NxtrConf,char(169),first,last)
      | end
  CorrSigAvlChkRev1 : Stateflow chart  TreatAsAtomicUnit=on
  Unit Delay : UnitDelay  SampleTime=-1  StateName=HwAgARollgCntPrev  StateMustResolveToSignalObject=on
      settings: AttributesFormatString=|
      | State Variable:
      | %<StateName>
  Unit Delay1 : UnitDelay  SampleTime=-1  StateName=HwAgAStallCntPrev  StateMustResolveToSignalObject=on
      settings: AttributesFormatString=|
      | State Variable:
      | %<StateName>
  HwAgAAvl : Outport
  wires:
  SigRollgCnt/1 -> CorrSigAvlChkRev1/1(SigRollgCnt), Unit Delay/1  "SigRollgCnt"
  SigQlfr/1 -> CorrSigAvlChkRev1/2(SigQlfr)  "SigQlfr"
  kMaxStallCnt/1 -> CorrSigAvlChkRev1/3(kMaxStallCnt)  "kMaxStallCnt"
  Unit Delay/1 -> CorrSigAvlChkRev1/4(LstRollgCnt)
  CorrSigAvlChkRev1/2(StallCntOutp) -> Unit Delay1/1
  Unit Delay1/1 -> CorrSigAvlChkRev1/5(LstStallCnt)
  CorrSigAvlChkRev1/1(SigAvl) -> HwAgAAvl/1

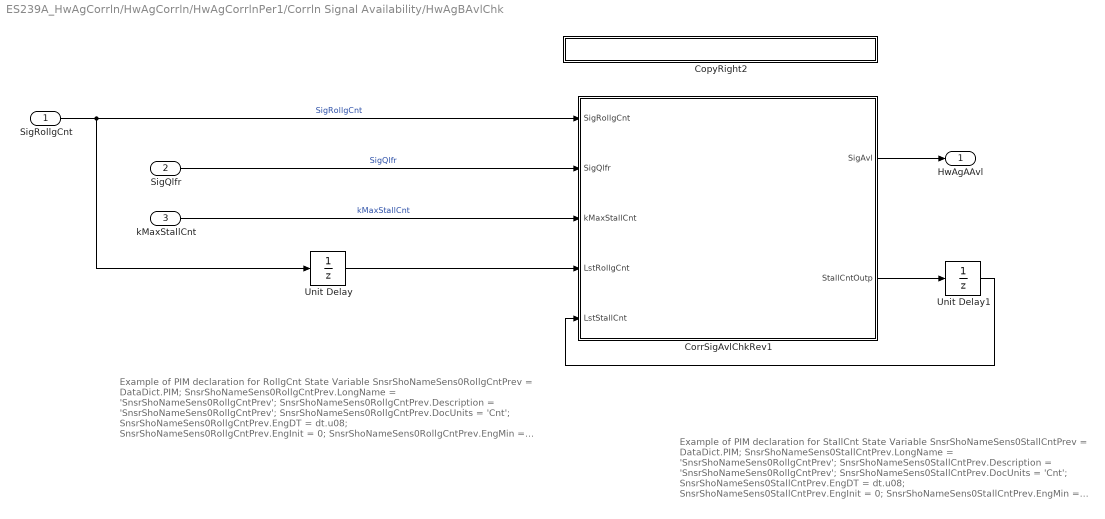
== system ES239A_HwAgCorrln/HwAgCorrln/HwAgCorrlnPer1/Corrln Signal Availability/HwAgBAvlChk ==
  note: Example of PIM declaration for StallCnt State Variable
      |
      | SnsrShoNameSens0StallCntPrev = DataDict.PIM;
      | SnsrShoNameSens0StallCntPrev.LongName = 'SnsrShoNameSens0RollgCntPrev';
      | SnsrShoNameSens0StallCntPrev.Description = 'SnsrShoNameSens0RollgCntPrev';
      | SnsrShoNameSens0StallCntPrev.DocUnits = 'Cnt';
      | SnsrShoNameSens0StallCntPrev.EngDT = dt.u08;
      | SnsrShoNameSens0StallCntPrev.EngInit = 0;
      | SnsrShoNameSens0StallCntPrev.EngMin = 0;
      | SnsrShoNameSens0StallCntPrev.EngMax = 255;
      |
      |
      | *********  Need different state variable for each instance of this  subsystem ********
  note: Example of PIM declaration for RollgCnt State Variable
      |
      | SnsrShoNameSens0RollgCntPrev = DataDict.PIM;
      | SnsrShoNameSens0RollgCntPrev.LongName = 'SnsrShoNameSens0RollgCntPrev';
      | SnsrShoNameSens0RollgCntPrev.Description = 'SnsrShoNameSens0RollgCntPrev';
      | SnsrShoNameSens0RollgCntPrev.DocUnits = 'Cnt';
      | SnsrShoNameSens0RollgCntPrev.EngDT = dt.u08;
      | SnsrShoNameSens0RollgCntPrev.EngInit = 0;
      | SnsrShoNameSens0RollgCntPrev.EngMin = 0;
      | SnsrShoNameSens0RollgCntPrev.EngMax = 255;
      |
      |
      | *********  Need different state variable for each instance of this  subsystem ********
  SigRollgCnt : Inport  OutDataTypeStr=uint8
  SigQlfr : Inport  Port=2  OutDataTypeStr=uint8
  kMaxStallCnt : Inport  Port=3  OutDataTypeStr=uint8
  CopyRight2 : Subsystem  Description=|  mask(Copyright Information){none=on}
      | Copyright info block.                                               
      |                                                                     
      | Place copyright information at the top of every subsystem in design.
      mask prompts: none "No parameters"
      mask help: Place copyright information at the top of every subsystem in design.
      mask Display:
      | NxtrConf = 'Nexteer Confidential';
      | 
      | sys = bdroot; %handle for the current model ("system")
      | first = get_param(sys,'Created');
      | first = first(end-3:end);  %year is last four digits
      | 
      | last = get_param(sys,'LastModifiedDate');
      | if isempty(last)
      |     last = datestr(now,'yyyy');
      | else
      |     last = last(end-3:end);
      | end
      | 
      | if strcmp(first,last)
      |     fprintf('%s -- Copyright %s Nexteer',NxtrConf,first)
      | else
      |     fprintf('%s -- %s%s- %s Nexteer',NxtrConf,char(169),first,last)
      | end
  CorrSigAvlChkRev1 : Stateflow chart  TreatAsAtomicUnit=on
  Unit Delay : UnitDelay  SampleTime=-1  StateName=HwAgBRollgCntPrev  StateMustResolveToSignalObject=on
      settings: AttributesFormatString=|
      | State Variable:
      | %<StateName>
  Unit Delay1 : UnitDelay  SampleTime=-1  StateName=HwAgBStallCntPrev  StateMustResolveToSignalObject=on
      settings: AttributesFormatString=|
      | State Variable:
      | %<StateName>
  HwAgAAvl : Outport
  wires:
  SigRollgCnt/1 -> CorrSigAvlChkRev1/1(SigRollgCnt), Unit Delay/1  "SigRollgCnt"
  SigQlfr/1 -> CorrSigAvlChkRev1/2(SigQlfr)  "SigQlfr"
  kMaxStallCnt/1 -> CorrSigAvlChkRev1/3(kMaxStallCnt)  "kMaxStallCnt"
  Unit Delay/1 -> CorrSigAvlChkRev1/4(LstRollgCnt)
  CorrSigAvlChkRev1/2(StallCntOutp) -> Unit Delay1/1
  Unit Delay1/1 -> CorrSigAvlChkRev1/5(LstStallCnt)
  CorrSigAvlChkRev1/1(SigAvl) -> HwAgAAvl/1

== system ES239A_HwAgCorrln/HwAgCorrln/HwAgCorrlnPer1/Correlation /FltInj_u08/CopyRight2 ==

== system ES239A_HwAgCorrln/HwAgCorrln/HwAgCorrlnPer1/Correlation /GetNtcSts/CopyRight2 ==

== system ES239A_HwAgCorrln/HwAgCorrln/HwAgCorrlnPer1/Correlation /Handwheel Angle Correlation Diagostic /CopyRight2 ==

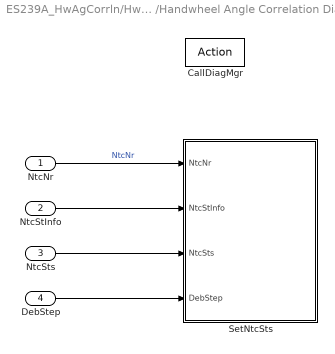
== system ES239A_HwAgCorrln/HwAgCorrln/HwAgCorrlnPer1/Correlation /Handwheel Angle Correlation Diagostic /SetNtcSts1 ==
  NtcNr : Inport
  NtcStInfo : Inport  Port=2
  NtcSts : Inport  Port=3
  DebStep : Inport  Port=4
  CallDiagMgr : ActionPort  ActionType=then
  SetNtcSts : Subsystem  RequirementInfo={} %GIDa_be7ee610_7ae4_4cb7_ad06_385711476099  TreatAsAtomicUnit=on
      settings: RTWSystemCode=Inline
  wires:
  NtcNr/1 -> SetNtcSts/1(NtcNr)  "NtcNr"
  NtcSts/1 -> SetNtcSts/3(NtcSts)
  DebStep/1 -> SetNtcSts/4(DebStep)
  NtcStInfo/1 -> SetNtcSts/2(NtcStInfo)

== system ES239A_HwAgCorrln/HwAgCorrln/HwAgCorrlnPer1/Correlation /Handwheel Angle Correlation Diagostic /SetNtcSts2 ==
  NtcNr : Inport
  NtcStInfo : Inport  Port=2
  NtcSts : Inport  Port=3
  DebStep : Inport  Port=4
  CallDiagMgr : ActionPort  ActionType=else
  SetNtcSts : Subsystem  RequirementInfo={} %GIDa_8741f13d_7e3e_49da_89b0_0d66569d73e0  TreatAsAtomicUnit=on
      settings: RTWSystemCode=Inline
  wires:
  NtcNr/1 -> SetNtcSts/1(NtcNr)  "NtcNr"
  NtcSts/1 -> SetNtcSts/3(NtcSts)
  DebStep/1 -> SetNtcSts/4(DebStep)
  NtcStInfo/1 -> SetNtcSts/2(NtcStInfo)

== system ES239A_HwAgCorrln/HwAgCorrln/HwAgCorrlnPer1/Corrln Signal Availability/HwAgAAvlChk/CopyRight2 ==

== system ES239A_HwAgCorrln/HwAgCorrln/HwAgCorrlnPer1/Corrln Signal Availability/HwAgBAvlChk/CopyRight2 ==

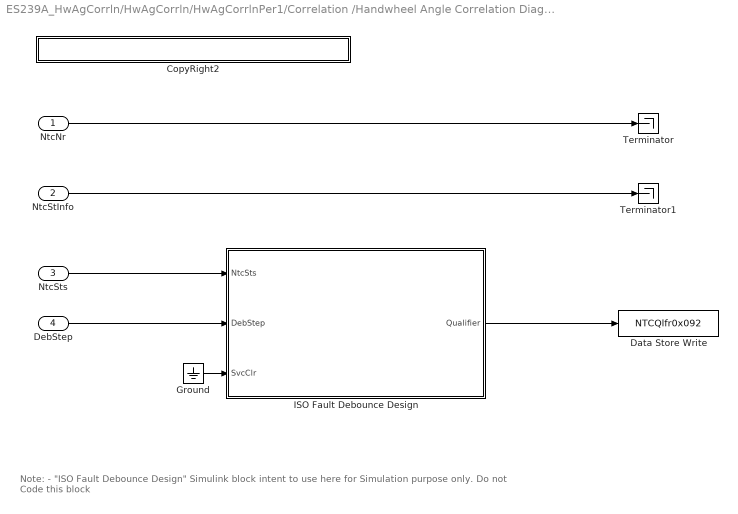
== system ES239A_HwAgCorrln/HwAgCorrln/HwAgCorrlnPer1/Correlation /Handwheel Angle Correlation Diagostic /SetNtcSts1/SetNtcSts ==
  note: Note:
      |
      | - "ISO Fault Debounce Design" Simulink block intent to use here for Simulation purpose only. Do not Code this block
  NtcNr : Inport
  NtcStInfo : Inport  Port=2
  NtcSts : Inport  Port=3
  DebStep : Inport  Port=4
  CopyRight2 : Subsystem  Description=|  mask(Copyright Information){none=on}
      | Copyright info block.                                               
      |                                                                     
      | Place copyright information at the top of every subsystem in design.
      mask prompts: none "No parameters"
      mask help: Place copyright information at the top of every subsystem in design.
      mask Display:
      | NxtrConf = 'Nexteer Confidential';
      | 
      | sys = bdroot; %handle for the current model ("system")
      | first = get_param(sys,'Created');
      | first = first(end-3:end);  %year is last four digits
      | 
      | last = get_param(sys,'LastModifiedDate');
      | if isempty(last)
      |     last = datestr(now,'yyyy');
      | else
      |     last = last(end-3:end);
      | end
      | 
      | if strcmp(first,last)
      |     fprintf('%s -- Copyright %s Nexteer',NxtrConf,first)
      | else
      |     fprintf('%s -- %s%s- %s Nexteer',NxtrConf,char(169),first,last)
      | end
  Data Store Write : DataStoreWrite  DataStoreName=NTCQlfr0x092
  Ground : Ground
  ISO Fault Debounce Design : Stateflow chart  TreatAsAtomicUnit=on
      settings: AttributesFormatString=|
      | Simulation Purpose Only.
      | Do Not Code this block
      | Diagnostic Manager Owns this requirement
  Terminator : Terminator
  Terminator1 : Terminator
  wires:
  NtcStInfo/1 -> Terminator1/1
  NtcNr/1 -> Terminator/1
  NtcSts/1 -> ISO Fault Debounce Design/1(NtcSts)
  DebStep/1 -> ISO Fault Debounce Design/2(DebStep)
  ISO Fault Debounce Design/1(Qualifier) -> Data Store Write/1
  Ground/1 -> ISO Fault Debounce Design/3(SvcClr)

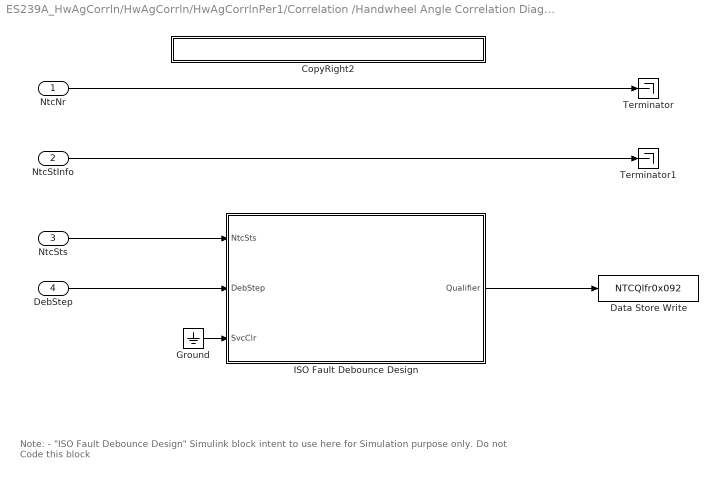
== system ES239A_HwAgCorrln/HwAgCorrln/HwAgCorrlnPer1/Correlation /Handwheel Angle Correlation Diagostic /SetNtcSts2/SetNtcSts ==
  note: Note:
      |
      | - "ISO Fault Debounce Design" Simulink block intent to use here for Simulation purpose only. Do not Code this block
  NtcNr : Inport
  NtcStInfo : Inport  Port=2
  NtcSts : Inport  Port=3
  DebStep : Inport  Port=4
  CopyRight2 : Subsystem  Description=|  mask(Copyright Information){none=on}
      | Copyright info block.                                               
      |                                                                     
      | Place copyright information at the top of every subsystem in design.
      mask prompts: none "No parameters"
      mask help: Place copyright information at the top of every subsystem in design.
      mask Display:
      | NxtrConf = 'Nexteer Confidential';
      | 
      | sys = bdroot; %handle for the current model ("system")
      | first = get_param(sys,'Created');
      | first = first(end-3:end);  %year is last four digits
      | 
      | last = get_param(sys,'LastModifiedDate');
      | if isempty(last)
      |     last = datestr(now,'yyyy');
      | else
      |     last = last(end-3:end);
      | end
      | 
      | if strcmp(first,last)
      |     fprintf('%s -- Copyright %s Nexteer',NxtrConf,first)
      | else
      |     fprintf('%s -- %s%s- %s Nexteer',NxtrConf,char(169),first,last)
      | end
  Data Store Write : DataStoreWrite  DataStoreName=NTCQlfr0x092
  Ground : Ground
  ISO Fault Debounce Design : Stateflow chart  TreatAsAtomicUnit=on
      settings: AttributesFormatString=|
      | Simulation Purpose Only.
      | Do Not Code this block
      | Diagnostic Manager Owns this requirement
  Terminator : Terminator
  Terminator1 : Terminator
  wires:
  NtcStInfo/1 -> Terminator1/1
  NtcNr/1 -> Terminator/1
  NtcSts/1 -> ISO Fault Debounce Design/1(NtcSts)
  DebStep/1 -> ISO Fault Debounce Design/2(DebStep)
  ISO Fault Debounce Design/1(Qualifier) -> Data Store Write/1
  Ground/1 -> ISO Fault Debounce Design/3(SvcClr)

== system ES239A_HwAgCorrln/HwAgCorrln/HwAgCorrlnPer1/Correlation /Handwheel Angle Correlation Diagostic /SetNtcSts1/SetNtcSts/CopyRight2 ==

== system ES239A_HwAgCorrln/HwAgCorrln/HwAgCorrlnPer1/Correlation /Handwheel Angle Correlation Diagostic /SetNtcSts2/SetNtcSts/CopyRight2 ==

== stateflow chart ES239A_HwAgCorrln/HwAgCorrln/HwAgCorrlnPer1/Corrln Signal Availability/HwAgBAvlChk/CorrSigAvlChkRev1 ==
  note: SigAvl
      | False = 0
      | Pass = 1
  note: SigQlfr
      | 0 = No Result
      | 1 = Pass
      | 2 = Fail
  (default) -> (junction 2)
  (junction 2) -> (junction 4) [order 1] : [SigRollgCnt ==LstRollgCnt]
  (junction 4) -> (junction 7) [order 2] : {
      | StallCntOutp = LstStallCnt +1;
      | }
  (junction 2) -> (junction 3) [order 2]
  (junction 4) -> (junction 7) [order 1] : [LstStallCnt == 255]
      | {
      | StallCntOutp = 255;
      | }
  (junction 3) -> (junction 7) : {
      | StallCntOutp = 0;
      | }
  (junction 7) -> (junction 10)
  (junction 10) -> (junction 12) [order 1] : [StallCntOutp >=kMaxStallCnt]
  (junction 10) -> (junction 14) [order 2]
  (junction 12) -> (junction 17)
  (junction 14) -> (junction 17) [order 2]
  (junction 14) -> (junction 16) [order 1] : [SigQlfr<2]
  (junction 17) -> (junction 29) : {
      | SigAvl =0;
      | }
  (junction 16) -> (junction 29) : {
      | SigAvl = 1;
      | }
  data: SigRollgCnt input; SigQlfr input; kMaxStallCnt input; SigAvl output uint8; LstRollgCnt input uint8; LstStallCnt input uint8; StallCntOutp output uint8

== matlab function ES239A_HwAgCorrln/HwAgCorrln/HwAgCorrlnPer1/Correlation /Determine Correlation Status ==
  data: HwAgAAvl input boolean; HwAgBAvl input boolean; CorrlnSt output uint8; ImmedCorrlnOk input boolean; LongTermCorrlnOk input uint8
function CorrlnSt = fcn(HwAgAAvl, HwAgBAvl, ImmedCorrlnOk, LongTermCorrlnOk)

aVarTruthTableCondition_1 = false;
aVarTruthTableCondition_2 = false;
aVarTruthTableCondition_3 = false;
aVarTruthTableCondition_4 = false;



aVarTruthTableCondition_1 = logical(LongTermCorrlnOk < 2);


aVarTruthTableCondition_2 = logical(HwAgAAvl);


aVarTruthTableCondition_3 = logical(HwAgBAvl);


aVarTruthTableCondition_4 = logical(ImmedCorrlnOk);

if (aVarTruthTableCondition_1 && aVarTruthTableCondition_2 && aVarTruthTableCondition_3 && aVarTruthTableCondition_4)
    aFcnTruthTableAction_1();
elseif (aVarTruthTableCondition_1 && aVarTruthTableCondition_2 && aVarTruthTableCondition_3 && ~aVarTruthTableCondition_4)
    aFcnTruthTableAction_4();
elseif (~aVarTruthTableCondition_1 && aVarTruthTableCondition_2 && aVarTruthTableCondition_3)
    aFcnTruthTableAction_4();
elseif (~aVarTruthTableCondition_2 && ~aVarTruthTableCondition_3)
    aFcnTruthTableAction_4();
elseif (aVarTruthTableCondition_2 && ~aVarTruthTableCondition_3)
    aFcnTruthTableAction_3();
else % Default
    aFcnTruthTableAction_2();
end

function aFcnTruthTableAction_1()

% A and B are Both Usable

CorrlnSt = uint8(3);

function aFcnTruthTableAction_2()

% B Only is usable

CorrlnSt = uint8(2);

function aFcnTruthTableAction_3()

% A Only is usable

CorrlnSt = uint8(1);

function aFcnTruthTableAction_4()

% no Signals Usable

CorrlnSt = uint8(0);

== stateflow chart ES239A_HwAgCorrln/HwAgCorrln/HwAgCorrlnPer1/Correlation /Handwheel Angle Correlation Diagostic /SetNtcSts1/SetNtcSts/ISO Fault Debounce Design ==
  note: NTCSTS_PASSD           (0)
      | NTCSTS_FAILD             (1)
      | NTCSTS_PREPASSD   (2)
      | NTCSTS_PREFAILD     (3)
      |
      | SIGQLFR_NORES        (0)
      | SIGQLFR_PASSD         (1)
      | SIGQLFR_FAILD           (2)
  note: Pass Loop
  note: Fail Loop
  note: 
  (default) -> (junction 89)
  (junction 89) -> (junction 95) [order 1] : [NtcSts ==3]
  (junction 89) -> (junction 93) [order 2] : [NtcSts ==2]
  (junction 89) -> (junction 141) [order 3] : [NtcSts ==1]
      | { ErrAcc = 32767;
      | Qualifier =2;
      |  }
  (junction 89) -> (junction 141) [order 4] : [NtcSts ==0]
      | { ErrAcc = -32768;
      | Qualifier=1;
      | }
  (junction 95) -> (junction 103) [order 2]
  (junction 95) -> (junction 111) [order 1] : [ErrAcc <=0]
      | {ErrAcc = DebStep;}
  (junction 93) -> (junction 123) [order 2] : {
      | ErrAcc = ErrAcc - DebStep;
      | }
  (junction 93) -> (junction 123) [order 1] : [(ErrAcc - DebStep) <= -32768]
      | { ErrAcc = -32768;
      | Qualifier=1;
      | }
  (junction 103) -> (junction 111) [order 1] : [(ErrAcc + DebStep) <32767]
      | {ErrAcc = ErrAcc + DebStep;}
  (junction 103) -> (junction 111) [order 2] : {ErrAcc = 32767;
      | Qualifier =2;}
  (junction 123) -> (junction 141)
  (junction 111) -> (junction 141)
  (junction 141) -> (junction 159) [order 2] : {ErrAcc = 0;
      | Qualifier =0;
      | }
  (junction 141) -> (junction 159) [order 1] : [SvcClr ==0]
  data: NtcSts input Enum: NtcSts1; Qualifier output uint8; DebStep input uint16; ErrAcc local single; SvcClr input
